simulink model "six_plus_six_AcmsteeringV09_main"  (R2014a)
settings: Solver=FixedStepDiscrete  StartTime=0.0  StopTime=10.0  FixedStep=0.0005  RelTol=1e-3
InitFcn:
  | Veh_Par_wxt
values from neighbouring files (symbols this model uses):
  acc_spdctl = [0 100]    [Veh_Par_wxt.m]
  ag_thr = ecucoder_cal(ag_thr)    [Veh_Par_wxt.m]
  B = 1.8    [Veh_Par_wxt.m]
  bra_em = 100    [Veh_Par_wxt.m]
  bra_pre_gz2 = 100/3    (= 33.3333333333)    [Veh_Par_wxt.m]
  bra_pre_gz34 = 10/3    (= 3.33333333333)    [Veh_Par_wxt.m]
  bra_pre_yd = 10/2    (= 5)    [Veh_Par_wxt.m]
  brakepre_dem_data = [0 1 2 3 4 5 6 7 8 9 10]    [Veh_Par_wxt.m]
  brakeTrq_dem_data = [0 125 251 376 502 627 753 878 1004 1129 1255]    [Veh_Par_wxt.m]
  bratrq_max = 4*1255    (= 5020)    [Veh_Par_wxt.m]
  eff_tran = 0.9    [Veh_Par_wxt.m]
  ESP_switch = ecucoder_cal(ESP_switch)    [Veh_Par_wxt.m]
  G = Mass*g    (= 15696)    [Veh_Par_wxt.m]
  kd1 = ecucoder_cal(kd1)    [Veh_Par_wxt.m]
  kd2 = 0    [Veh_Par_wxt.m]
  ki1 = ecucoder_cal(ki1)    [Veh_Par_wxt.m]
  ki2 = 1    [Veh_Par_wxt.m]
  kp1 = ecucoder_cal(kp1)    [Veh_Par_wxt.m]
  kp2 = 300    [Veh_Par_wxt.m]
  L = L1+L2    (= 2.9)    [Veh_Par_wxt.m]
  premax = 100    [Veh_Par_wxt.m]
  Radius = 0.4572/2    (= 0.2286)    [Veh_Par_wxt.m]
  RC_switch = ecucoder_cal(RC_switch)    [Veh_Par_wxt.m]
  s_opt_yi = 0.15    [Veh_Par_wxt.m]
  s_opt_zhuan = 0.8    [Veh_Par_wxt.m]
  s_opt_zhuan_add = 0.05    [Veh_Par_wxt.m]
  s_opt_zhuan_table = [0.8 0.8 0.3 0.3]    [Veh_Par_wxt.m]
  spd_map_mot = [0 499.85 999.79 1500 2000 2500 3000 3500 4000 4500 4999.8 5999.8]    [Veh_Par_wxt.m]
  spd_spdctl = [0 500]    [Veh_Par_wxt.m]
  speed_thr_park = 5/3.6/Radius*tras_ratio*30/pi    (= 464.143899364)    [Veh_Par_wxt.m]
  TCS_switch = ecucoder_cal(TCS_switch)    [Veh_Par_wxt.m]
  tras_ratio = 8    [Veh_Par_wxt.m]
  trq_map_mot = [70.5 70.012 71.154 65.797 53.917 45.159 38.073 32.685 27.48 17.133 14.949 10.07]    [Veh_Par_wxt.m]
  trqmax_yd = 70.5    [Veh_Par_wxt.m]
  trqmax_zx = 70.5    [Veh_Par_wxt.m]
  trqmaxneg = -70.5    [Veh_Par_wxt.m]
  v_gain = 0.9    [Veh_Par_wxt.m]
  v_table = [0 5 20 100]    [Veh_Par_wxt.m]
  v_thr_park = 5    [Veh_Par_wxt.m]
  zhidong_bianmazhi = [-140000 750000]    [Veh_Par_wxt.m]
  zhidong_down = -140000    [Veh_Par_wxt.m]
  zhidong_up = 750000    [Veh_Par_wxt.m]
  zhidong_youmen = [0 100]    [Veh_Par_wxt.m]
  zhuanxiang_bianmazhi = [-400000 0 400000]    [Veh_Par_wxt.m]
  zhuanxiang_down = -400000    [Veh_Par_wxt.m]
  zhuanxiang_up = 400000    [Veh_Par_wxt.m]
  zhuanxiang_youmen = [-100 0 100]    [Veh_Par_wxt.m]
undefined symbols (not defined in the file or in its folder): ecucoder_acal, guzhang_lf, guzhang_lm, guzhang_lr, guzhang_rf, guzhang_rm, guzhang_rr, myFIS
libraries: simulink x979, ec5744lib x59, fuzblock x2
(part 3 of 26)

== system six_plus_six_AcmsteeringV09_main/Data_input/MCU2 ==
  In1 : Inport
  In2 : Inport  Port=2
  Trigger : TriggerPort  TriggerType=function-call  PortDimensions=1
  MCU2 : Subsystem
  MCU2_MotorStallingFault : Outport
  MCU2_UdcDetectionFault : Outport  Port=2
  MCU2_TempSensorFault : Outport  Port=3
  MCU2_ActiveDischargingFault : Outport  Port=4
  MCU2_ldcSensorFault : Outport  Port=5
  MCU2_luSensorFault : Outport  Port=6
  MCU2_lvSensorFault : Outport  Port=7
  MCU2_FaultLevel : Outport  Port=8
  MCU2_Controllerload : Outport  Port=9
  MCU2_CanCommunicationFault : Outport  Port=10
  MCU2_MemoryFault : Outport  Port=11
  MCU2_DownratingFault : Outport  Port=12
  MCU2_IGBTFault : Outport  Port=13
  MCU2_MotorOverTemp : Outport  Port=14
  MCU2_ControllerOverTemp : Outport  Port=15
  MCU2_MotorOverSpeed : Outport  Port=16
  MCU2_RotaryInverterFault : Outport  Port=17
  MCU2_UnderVoltage : Outport  Port=18
  MCU2_OverVoltage : Outport  Port=19
  MCU2_MotorOverLoad : Outport  Port=20
  wires:
  MCU2/1(MCU2_MotorStallingFault_Out) -> MCU2_MotorStallingFault/1
  MCU2/7(MCU2_IvSensorFault_Out) -> MCU2_lvSensorFault/1
  MCU2/4(MCU2_ActieDischargingFault_Out) -> MCU2_ActiveDischargingFault/1
  MCU2/12(MCU2_DownratingFault_Out) -> MCU2_DownratingFault/1
  MCU2/13(MCU2_IGBTFault_Out) -> MCU2_IGBTFault/1
  MCU2/3(MCU2_TempSensorFault_Out) -> MCU2_TempSensorFault/1
  MCU2/10(MCU2_CanCommunicationFault_Out) -> MCU2_CanCommunicationFault/1
  MCU2/11(MCU2_MemoryFault_Out) -> MCU2_MemoryFault/1
  MCU2/14(MCU2_MotorOverTemp_Out) -> MCU2_MotorOverTemp/1
  MCU2/2(MCU2_UdcDetectionFault_Out) -> MCU2_UdcDetectionFault/1
  MCU2/5(MCU2_IdcSensorFault_Out) -> MCU2_ldcSensorFault/1
  In2/1 -> MCU2/1(input)
  In1/1 -> MCU2/Enable
  MCU2/6(MCU2_IuSensorFault_Out) -> MCU2_luSensorFault/1
  MCU2/8(MCU2_FaultLevel_Out) -> MCU2_FaultLevel/1
  MCU2/9(MCU2_ControllerOverload_Out) -> MCU2_Controllerload/1
  MCU2/20(MCU2_MotorOverLoad_Out) -> MCU2_MotorOverLoad/1
  MCU2/18(MCU2_UnderVoltage_Out) -> MCU2_UnderVoltage/1
  MCU2/19(MCU2_OverVoltage_Out) -> MCU2_OverVoltage/1
  MCU2/15(MCU2_ControllerOverTemp_Out) -> MCU2_ControllerOverTemp/1
  MCU2/16(MCU2_MotorOverSpeed_Out) -> MCU2_MotorOverSpeed/1
  MCU2/17(MCU2_RotaryInverterFault_Out) -> MCU2_RotaryInverterFault/1

== matlab function six_plus_six_AcmsteeringV09_main/Data_input/3/Enabled Subsystem/MATLAB Function1 ==
  data: current_in input; current_out output
function current_out = motec_current(current_in)
    if current_in>32768
        current_out=current_in-65535;
    else
        current_out=current_in;
    end
end

== matlab function six_plus_six_AcmsteeringV09_main/MainControl/mode_control/backward/backward/Brake/HeartBeat2 ==
  data: life_pre input; life output
function life = fcn(life_pre)
%#codegen
life=single(life_pre+1);
if life>255
    life=single(0);
end
end

== matlab function six_plus_six_AcmsteeringV09_main/MainControl/mode_control/backward/backward/Drive/左右侧电机分配及功率限制/MATLAB Function ==
  data: trqlim_l input; trq_dem_l output; trq_dem_r output; trq_dem_l1 input; trqlim_r input; trq_dem_r1 input; delta_T_dem input
function [trq_dem_l,trq_dem_r] = fcn(trqlim_l,trq_dem_l1,trqlim_r,trq_dem_r1,delta_T_dem)
%#codegen
if trq_dem_l1==trqlim_l
    trq_dem_l=single(trq_dem_l1);
    trq_dem_r=single(trq_dem_l1+delta_T_dem);%这时候加的是负值
elseif trq_dem_r1==trqlim_r
    trq_dem_l=single(trq_dem_r1-delta_T_dem);
    trq_dem_r=single(trq_dem_r1);
    
else
    trq_dem_l=single(trq_dem_l1);
    trq_dem_r=single(trq_dem_r1);
end
% trq_dem_l=single(max(0,trq_dem_l));%限一下最小值，不要小于0
% trq_dem_r=single(max(0,trq_dem_r));
trq_dem_l=single(max(-trqlim_l,trq_dem_l));%小转向半径下，内侧履带是可能输出负转矩的，从地面吸收功率，给外侧，所以不能限到0，限到最大电机外特性负值
trq_dem_r=single(max(-trqlim_r,trq_dem_r));
end

== matlab function six_plus_six_AcmsteeringV09_main/MainControl/mode_control/forward/forward/Brake/HeartBeat ==
  data: life_pre input; life output
function life = fcn(life_pre)
%#codegen
life=single(life_pre+1);
if life>255
    life=single(0);
end
end

== matlab function six_plus_six_AcmsteeringV09_main/MainControl/mode_control/center_steer/center_steer/HeartBeat4 ==
  data: life_pre input; life output
function life = fcn(life_pre)
%#codegen
life=single(life_pre+1);
if life>255
    life=single(0);
end
end

== matlab function six_plus_six_AcmsteeringV09_main/MainControl/mode_control/emergency_stop/emergency_stop/HeartBeat5 ==
  data: life_pre input; life output
function life = fcn(life_pre)
%#codegen
life=single(life_pre+1);
if life>255
    life=single(0);
end
end

== matlab function six_plus_six_AcmsteeringV09_main/MainControl/mode_control/neutral/neutral/HeartBeat5 ==
  data: life_pre input; life output
function life = fcn(life_pre)
%#codegen
life=single(life_pre+1);
if life>255
    life=single(0);
end
end

== matlab function six_plus_six_AcmsteeringV09_main/MainControl/mode_control/backward/backward/Drive/驱动防滑控制TCS/直行TCS/直行/MATLAB Function2 ==
  data: s_act_rf input; flag_rf output; s_opt_zhuan input; s_opt_zhuan_add input; flag_rf_pre input int8
function flag_rf = fcn(s_act_rf,s_opt_zhuan,s_opt_zhuan_add,flag_rf_pre)
%#codegen
if s_act_rf>s_opt_zhuan+s_opt_zhuan_add
    flag_rf=int8(1);
elseif s_act_rf<s_opt_zhuan
    flag_rf =int8(0);
else
    flag_rf=int8(flag_rf_pre);
end
end

== matlab function six_plus_six_AcmsteeringV09_main/Data_input/5/Enabled Subsystem/MATLAB Function ==
  data: data1 input; y output; data2 input; data3 input; data4 input
function y = fcn(data1,data2,data3,data4)
%#codegen
y1=data4*256^3+data3*256^2+data2*256+data1;
y=typecast(uint32(y1),'single');
end
% y = u;

== matlab function six_plus_six_AcmsteeringV09_main/Data_input/7/Enabled
Subsystem/MATLAB Function1 ==
  data: data1 input; y output; data2 input; data3 input; data4 input
function y = fcn(data1,data2,data3,data4)
%#codegen
y1=data4*256^3+data3*256^2+data2*256+data1;
y=typecast(uint32(y1),'single');
end
% y = u;

== matlab function six_plus_six_AcmsteeringV09_main/InputSignalProcess/MATLAB Function1 ==
  data: Xangularrate input; Yangularrate input; Zangularrate input; Xacceleration input; Yacceleration input; Zacceleration input; Xangularrate1 output; Yangularrate1 output; Zangularrate1 output; Xacceleration1 output; Yacceleration1 output; Zacceleration1 output; NorthSpd1 output; SkySpd1 output; EastSpd1 output; Altitude1 output; Longitude1 output; Latitude1 output; Rolling1 output; Heading1 output; Pitching1 output; NorthSpd input; SkySpd input; Xspd output; EastSpd input; Altitude input; Longitude input; Latitude input; Rolling input; Heading input; Yspd output; Pitching input
function [Xangularrate1,Yangularrate1,Zangularrate1,Xacceleration1,Yacceleration1,Zacceleration1,NorthSpd1,SkySpd1,EastSpd1,Altitude1,Longitude1,Latitude1,Rolling1,Heading1,Pitching1,Xspd,Yspd] = fcn(Xangularrate,Yangularrate,Zangularrate,Xacceleration,Yacceleration,Zacceleration,NorthSpd,SkySpd,EastSpd,Altitude,Longitude,Latitude,Rolling,Heading,Pitching)
%#codegen
Xangularrate1=Xangularrate;
Yangularrate1=-Zangularrate;
Zangularrate1=-Yangularrate;
Xacceleration1=Xacceleration;
Yacceleration1=-Zacceleration;
Zacceleration1=-Yacceleration;
NorthSpd1=NorthSpd;
SkySpd1=SkySpd;
EastSpd1=EastSpd;
Altitude1=Altitude;
Longitude1=Longitude;
Latitude1=Latitude;
Rolling1=Rolling;
Heading1=Heading;
Pitching1=Pitching;
Xspd=NorthSpd*cos(Heading/180*pi)-EastSpd*sin(Heading/180*pi);
Yspd=-(NorthSpd*sin(Heading/180*pi)+EastSpd*cos(Heading/180*pi));
end
% y = u;

== system six_plus_six_AcmsteeringV09_main/Data_input/MCU2_1 ==
  In1 : Inport
  In2 : Inport  Port=2
  Trigger : TriggerPort  TriggerType=function-call  PortDimensions=1
  MCU2 : Subsystem
  MCU2_MotorStallingFault : Outport
  MCU2_UdcDetectionFault : Outport  Port=2
  MCU2_TempSensorFault : Outport  Port=3
  MCU2_ActiveDischargingFault : Outport  Port=4
  MCU2_ldcSensorFault : Outport  Port=5
  MCU2_luSensorFault : Outport  Port=6
  MCU2_lvSensorFault : Outport  Port=7
  MCU2_FaultLevel : Outport  Port=8
  MCU2_Controllerload : Outport  Port=9
  MCU2_CanCommunicationFault : Outport  Port=10
  MCU2_MemoryFault : Outport  Port=11
  MCU2_DownratingFault : Outport  Port=12
  MCU2_IGBTFault : Outport  Port=13
  MCU2_MotorOverTemp : Outport  Port=14
  MCU2_ControllerOverTemp : Outport  Port=15
  MCU2_MotorOverSpeed : Outport  Port=16
  MCU2_RotaryInverterFault : Outport  Port=17
  MCU2_UnderVoltage : Outport  Port=18
  MCU2_OverVoltage : Outport  Port=19
  MCU2_MotorOverLoad : Outport  Port=20
  wires:
  MCU2/1(MCU2_MotorStallingFault_Out) -> MCU2_MotorStallingFault/1
  MCU2/7(MCU2_IvSensorFault_Out) -> MCU2_lvSensorFault/1
  MCU2/4(MCU2_ActieDischargingFault_Out) -> MCU2_ActiveDischargingFault/1
  MCU2/12(MCU2_DownratingFault_Out) -> MCU2_DownratingFault/1
  MCU2/13(MCU2_IGBTFault_Out) -> MCU2_IGBTFault/1
  MCU2/3(MCU2_TempSensorFault_Out) -> MCU2_TempSensorFault/1
  MCU2/10(MCU2_CanCommunicationFault_Out) -> MCU2_CanCommunicationFault/1
  MCU2/11(MCU2_MemoryFault_Out) -> MCU2_MemoryFault/1
  MCU2/14(MCU2_MotorOverTemp_Out) -> MCU2_MotorOverTemp/1
  MCU2/2(MCU2_UdcDetectionFault_Out) -> MCU2_UdcDetectionFault/1
  MCU2/5(MCU2_IdcSensorFault_Out) -> MCU2_ldcSensorFault/1
  In2/1 -> MCU2/1(input)
  In1/1 -> MCU2/Enable
  MCU2/6(MCU2_IuSensorFault_Out) -> MCU2_luSensorFault/1
  MCU2/8(MCU2_FaultLevel_Out) -> MCU2_FaultLevel/1
  MCU2/9(MCU2_ControllerOverload_Out) -> MCU2_Controllerload/1
  MCU2/20(MCU2_MotorOverLoad_Out) -> MCU2_MotorOverLoad/1
  MCU2/18(MCU2_UnderVoltage_Out) -> MCU2_UnderVoltage/1
  MCU2/19(MCU2_OverVoltage_Out) -> MCU2_OverVoltage/1
  MCU2/15(MCU2_ControllerOverTemp_Out) -> MCU2_ControllerOverTemp/1
  MCU2/16(MCU2_MotorOverSpeed_Out) -> MCU2_MotorOverSpeed/1
  MCU2/17(MCU2_RotaryInverterFault_Out) -> MCU2_RotaryInverterFault/1

== system six_plus_six_AcmsteeringV09_main/Data_input/MCU2_2 ==
  In1 : Inport
  In2 : Inport  Port=2
  Trigger : TriggerPort  TriggerType=function-call  PortDimensions=1
  MCU2 : Subsystem
  MCU2_MotorStallingFault : Outport
  MCU2_UdcDetectionFault : Outport  Port=2
  MCU2_TempSensorFault : Outport  Port=3
  MCU2_ActiveDischargingFault : Outport  Port=4
  MCU2_ldcSensorFault : Outport  Port=5
  MCU2_luSensorFault : Outport  Port=6
  MCU2_lvSensorFault : Outport  Port=7
  MCU2_FaultLevel : Outport  Port=8
  MCU2_Controllerload : Outport  Port=9
  MCU2_CanCommunicationFault : Outport  Port=10
  MCU2_MemoryFault : Outport  Port=11
  MCU2_DownratingFault : Outport  Port=12
  MCU2_IGBTFault : Outport  Port=13
  MCU2_MotorOverTemp : Outport  Port=14
  MCU2_ControllerOverTemp : Outport  Port=15
  MCU2_MotorOverSpeed : Outport  Port=16
  MCU2_RotaryInverterFault : Outport  Port=17
  MCU2_UnderVoltage : Outport  Port=18
  MCU2_OverVoltage : Outport  Port=19
  MCU2_MotorOverLoad : Outport  Port=20
  wires:
  MCU2/1(MCU2_MotorStallingFault_Out) -> MCU2_MotorStallingFault/1
  MCU2/7(MCU2_IvSensorFault_Out) -> MCU2_lvSensorFault/1
  MCU2/4(MCU2_ActieDischargingFault_Out) -> MCU2_ActiveDischargingFault/1
  MCU2/12(MCU2_DownratingFault_Out) -> MCU2_DownratingFault/1
  MCU2/13(MCU2_IGBTFault_Out) -> MCU2_IGBTFault/1
  MCU2/3(MCU2_TempSensorFault_Out) -> MCU2_TempSensorFault/1
  MCU2/10(MCU2_CanCommunicationFault_Out) -> MCU2_CanCommunicationFault/1
  MCU2/11(MCU2_MemoryFault_Out) -> MCU2_MemoryFault/1
  MCU2/14(MCU2_MotorOverTemp_Out) -> MCU2_MotorOverTemp/1
  MCU2/2(MCU2_UdcDetectionFault_Out) -> MCU2_UdcDetectionFault/1
  MCU2/5(MCU2_IdcSensorFault_Out) -> MCU2_ldcSensorFault/1
  In2/1 -> MCU2/1(input)
  In1/1 -> MCU2/Enable
  MCU2/6(MCU2_IuSensorFault_Out) -> MCU2_luSensorFault/1
  MCU2/8(MCU2_FaultLevel_Out) -> MCU2_FaultLevel/1
  MCU2/9(MCU2_ControllerOverload_Out) -> MCU2_Controllerload/1
  MCU2/20(MCU2_MotorOverLoad_Out) -> MCU2_MotorOverLoad/1
  MCU2/18(MCU2_UnderVoltage_Out) -> MCU2_UnderVoltage/1
  MCU2/19(MCU2_OverVoltage_Out) -> MCU2_OverVoltage/1
  MCU2/15(MCU2_ControllerOverTemp_Out) -> MCU2_ControllerOverTemp/1
  MCU2/16(MCU2_MotorOverSpeed_Out) -> MCU2_MotorOverSpeed/1
  MCU2/17(MCU2_RotaryInverterFault_Out) -> MCU2_RotaryInverterFault/1

== system six_plus_six_AcmsteeringV09_main/Data_input/MCU2_3 ==
  In1 : Inport
  In2 : Inport  Port=2
  Trigger : TriggerPort  TriggerType=function-call  PortDimensions=1
  MCU2 : Subsystem
  MCU2_MotorStallingFault : Outport
  MCU2_UdcDetectionFault : Outport  Port=2
  MCU2_TempSensorFault : Outport  Port=3
  MCU2_ActiveDischargingFault : Outport  Port=4
  MCU2_ldcSensorFault : Outport  Port=5
  MCU2_luSensorFault : Outport  Port=6
  MCU2_lvSensorFault : Outport  Port=7
  MCU2_FaultLevel : Outport  Port=8
  MCU2_Controllerload : Outport  Port=9
  MCU2_CanCommunicationFault : Outport  Port=10
  MCU2_MemoryFault : Outport  Port=11
  MCU2_DownratingFault : Outport  Port=12
  MCU2_IGBTFault : Outport  Port=13
  MCU2_MotorOverTemp : Outport  Port=14
  MCU2_ControllerOverTemp : Outport  Port=15
  MCU2_MotorOverSpeed : Outport  Port=16
  MCU2_RotaryInverterFault : Outport  Port=17
  MCU2_UnderVoltage : Outport  Port=18
  MCU2_OverVoltage : Outport  Port=19
  MCU2_MotorOverLoad : Outport  Port=20
  wires:
  MCU2/1(MCU2_MotorStallingFault_Out) -> MCU2_MotorStallingFault/1
  MCU2/7(MCU2_IvSensorFault_Out) -> MCU2_lvSensorFault/1
  MCU2/4(MCU2_ActieDischargingFault_Out) -> MCU2_ActiveDischargingFault/1
  MCU2/12(MCU2_DownratingFault_Out) -> MCU2_DownratingFault/1
  MCU2/13(MCU2_IGBTFault_Out) -> MCU2_IGBTFault/1
  MCU2/3(MCU2_TempSensorFault_Out) -> MCU2_TempSensorFault/1
  MCU2/10(MCU2_CanCommunicationFault_Out) -> MCU2_CanCommunicationFault/1
  MCU2/11(MCU2_MemoryFault_Out) -> MCU2_MemoryFault/1
  MCU2/14(MCU2_MotorOverTemp_Out) -> MCU2_MotorOverTemp/1
  MCU2/2(MCU2_UdcDetectionFault_Out) -> MCU2_UdcDetectionFault/1
  MCU2/5(MCU2_IdcSensorFault_Out) -> MCU2_ldcSensorFault/1
  In2/1 -> MCU2/1(input)
  In1/1 -> MCU2/Enable
  MCU2/6(MCU2_IuSensorFault_Out) -> MCU2_luSensorFault/1
  MCU2/8(MCU2_FaultLevel_Out) -> MCU2_FaultLevel/1
  MCU2/9(MCU2_ControllerOverload_Out) -> MCU2_Controllerload/1
  MCU2/20(MCU2_MotorOverLoad_Out) -> MCU2_MotorOverLoad/1
  MCU2/18(MCU2_UnderVoltage_Out) -> MCU2_UnderVoltage/1
  MCU2/19(MCU2_OverVoltage_Out) -> MCU2_OverVoltage/1
  MCU2/15(MCU2_ControllerOverTemp_Out) -> MCU2_ControllerOverTemp/1
  MCU2/16(MCU2_MotorOverSpeed_Out) -> MCU2_MotorOverSpeed/1
  MCU2/17(MCU2_RotaryInverterFault_Out) -> MCU2_RotaryInverterFault/1

== system six_plus_six_AcmsteeringV09_main/Data_input/MCU2_4 ==
  In1 : Inport
  In2 : Inport  Port=2
  Trigger : TriggerPort  TriggerType=function-call  PortDimensions=1
  MCU2 : Subsystem
  MCU2_MotorStallingFault : Outport
  MCU2_UdcDetectionFault : Outport  Port=2
  MCU2_TempSensorFault : Outport  Port=3
  MCU2_ActiveDischargingFault : Outport  Port=4
  MCU2_ldcSensorFault : Outport  Port=5
  MCU2_luSensorFault : Outport  Port=6
  MCU2_lvSensorFault : Outport  Port=7
  MCU2_FaultLevel : Outport  Port=8
  MCU2_Controllerload : Outport  Port=9
  MCU2_CanCommunicationFault : Outport  Port=10
  MCU2_MemoryFault : Outport  Port=11
  MCU2_DownratingFault : Outport  Port=12
  MCU2_IGBTFault : Outport  Port=13
  MCU2_MotorOverTemp : Outport  Port=14
  MCU2_ControllerOverTemp : Outport  Port=15
  MCU2_MotorOverSpeed : Outport  Port=16
  MCU2_RotaryInverterFault : Outport  Port=17
  MCU2_UnderVoltage : Outport  Port=18
  MCU2_OverVoltage : Outport  Port=19
  MCU2_MotorOverLoad : Outport  Port=20
  wires:
  MCU2/1(MCU2_MotorStallingFault_Out) -> MCU2_MotorStallingFault/1
  MCU2/7(MCU2_IvSensorFault_Out) -> MCU2_lvSensorFault/1
  MCU2/4(MCU2_ActieDischargingFault_Out) -> MCU2_ActiveDischargingFault/1
  MCU2/12(MCU2_DownratingFault_Out) -> MCU2_DownratingFault/1
  MCU2/13(MCU2_IGBTFault_Out) -> MCU2_IGBTFault/1
  MCU2/3(MCU2_TempSensorFault_Out) -> MCU2_TempSensorFault/1
  MCU2/10(MCU2_CanCommunicationFault_Out) -> MCU2_CanCommunicationFault/1
  MCU2/11(MCU2_MemoryFault_Out) -> MCU2_MemoryFault/1
  MCU2/14(MCU2_MotorOverTemp_Out) -> MCU2_MotorOverTemp/1
  MCU2/2(MCU2_UdcDetectionFault_Out) -> MCU2_UdcDetectionFault/1
  MCU2/5(MCU2_IdcSensorFault_Out) -> MCU2_ldcSensorFault/1
  In2/1 -> MCU2/1(input)
  In1/1 -> MCU2/Enable
  MCU2/6(MCU2_IuSensorFault_Out) -> MCU2_luSensorFault/1
  MCU2/8(MCU2_FaultLevel_Out) -> MCU2_FaultLevel/1
  MCU2/9(MCU2_ControllerOverload_Out) -> MCU2_Controllerload/1
  MCU2/20(MCU2_MotorOverLoad_Out) -> MCU2_MotorOverLoad/1
  MCU2/18(MCU2_UnderVoltage_Out) -> MCU2_UnderVoltage/1
  MCU2/19(MCU2_OverVoltage_Out) -> MCU2_OverVoltage/1
  MCU2/15(MCU2_ControllerOverTemp_Out) -> MCU2_ControllerOverTemp/1
  MCU2/16(MCU2_MotorOverSpeed_Out) -> MCU2_MotorOverSpeed/1
  MCU2/17(MCU2_RotaryInverterFault_Out) -> MCU2_RotaryInverterFault/1

== system six_plus_six_AcmsteeringV09_main/Data_input/MCU2_5 ==
  In1 : Inport
  In2 : Inport  Port=2
  Trigger : TriggerPort  TriggerType=function-call  PortDimensions=1
  MCU2 : Subsystem
  MCU2_MotorStallingFault : Outport
  MCU2_UdcDetectionFault : Outport  Port=2
  MCU2_TempSensorFault : Outport  Port=3
  MCU2_ActiveDischargingFault : Outport  Port=4
  MCU2_ldcSensorFault : Outport  Port=5
  MCU2_luSensorFault : Outport  Port=6
  MCU2_lvSensorFault : Outport  Port=7
  MCU2_FaultLevel : Outport  Port=8
  MCU2_Controllerload : Outport  Port=9
  MCU2_CanCommunicationFault : Outport  Port=10
  MCU2_MemoryFault : Outport  Port=11
  MCU2_DownratingFault : Outport  Port=12
  MCU2_IGBTFault : Outport  Port=13
  MCU2_MotorOverTemp : Outport  Port=14
  MCU2_ControllerOverTemp : Outport  Port=15
  MCU2_MotorOverSpeed : Outport  Port=16
  MCU2_RotaryInverterFault : Outport  Port=17
  MCU2_UnderVoltage : Outport  Port=18
  MCU2_OverVoltage : Outport  Port=19
  MCU2_MotorOverLoad : Outport  Port=20
  wires:
  MCU2/1(MCU2_MotorStallingFault_Out) -> MCU2_MotorStallingFault/1
  MCU2/7(MCU2_IvSensorFault_Out) -> MCU2_lvSensorFault/1
  MCU2/4(MCU2_ActieDischargingFault_Out) -> MCU2_ActiveDischargingFault/1
  MCU2/12(MCU2_DownratingFault_Out) -> MCU2_DownratingFault/1
  MCU2/13(MCU2_IGBTFault_Out) -> MCU2_IGBTFault/1
  MCU2/3(MCU2_TempSensorFault_Out) -> MCU2_TempSensorFault/1
  MCU2/10(MCU2_CanCommunicationFault_Out) -> MCU2_CanCommunicationFault/1
  MCU2/11(MCU2_MemoryFault_Out) -> MCU2_MemoryFault/1
  MCU2/14(MCU2_MotorOverTemp_Out) -> MCU2_MotorOverTemp/1
  MCU2/2(MCU2_UdcDetectionFault_Out) -> MCU2_UdcDetectionFault/1
  MCU2/5(MCU2_IdcSensorFault_Out) -> MCU2_ldcSensorFault/1
  In2/1 -> MCU2/1(input)
  In1/1 -> MCU2/Enable
  MCU2/6(MCU2_IuSensorFault_Out) -> MCU2_luSensorFault/1
  MCU2/8(MCU2_FaultLevel_Out) -> MCU2_FaultLevel/1
  MCU2/9(MCU2_ControllerOverload_Out) -> MCU2_Controllerload/1
  MCU2/20(MCU2_MotorOverLoad_Out) -> MCU2_MotorOverLoad/1
  MCU2/18(MCU2_UnderVoltage_Out) -> MCU2_UnderVoltage/1
  MCU2/19(MCU2_OverVoltage_Out) -> MCU2_OverVoltage/1
  MCU2/15(MCU2_ControllerOverTemp_Out) -> MCU2_ControllerOverTemp/1
  MCU2/16(MCU2_MotorOverSpeed_Out) -> MCU2_MotorOverSpeed/1
  MCU2/17(MCU2_RotaryInverterFault_Out) -> MCU2_RotaryInverterFault/1

== system six_plus_six_AcmsteeringV09_main/Data_input/RemoteControl1 ==
  In1 : Inport
  In2 : Inport  Port=2
  Trigger : TriggerPort  TriggerType=function-call  PortDimensions=1
  Yaokong2 : Subsystem
  SH : Outport
  SE : Outport  Port=2
  SD : Outport  Port=3
  SA : Outport  Port=4
  LIFEspan : Outport  Port=5
  wires:
  Yaokong2/2(SE_Out) -> SE/1
  Yaokong2/3(SD_Out) -> SD/1
  Yaokong2/4(SA_Out) -> SA/1
  In2/1 -> Yaokong2/1(input)
  In1/1 -> Yaokong2/Enable
  Yaokong2/1(SH_Out) -> SH/1
  Yaokong2/5(LIFEspan_Out) -> LIFEspan/1

== system six_plus_six_AcmsteeringV09_main/Data_input/RemoteControl2 ==
  In1 : Inport
  In2 : Inport  Port=2
  Trigger : TriggerPort  TriggerType=function-call  PortDimensions=1
  Yaokong1 : Subsystem
  Rightstick_updown : Outport
  Rightstick_leftright : Outport  Port=2
  Leftstick_updown : Outport  Port=3
  Leftstick_leftright : Outport  Port=4
  wires:
  In1/1 -> Yaokong1/Enable
  In2/1 -> Yaokong1/1(input)
  Yaokong1/1(Rightstick_updown_Out) -> Rightstick_updown/1
  Yaokong1/2(Rightstick_leftright_Out) -> Rightstick_leftright/1
  Yaokong1/3(Leftstick_updown_Out) -> Leftstick_updown/1
  Yaokong1/4(Leftstick_leftright_Out) -> Leftstick_leftright/1

== system six_plus_six_AcmsteeringV09_main/MainControl/mode_control ==
  mode_dem_out : Inport
  Signals : Inport  Port=2
  Multiport Switch : MultiPortSwitch  DataPortOrder=Zero-based contiguous  Inputs=6
  Park : Subsystem  TreatAsAtomicUnit=on
  Switch Case : SwitchCase  CaseConditions={0,1,2,3,4,5}  ShowDefaultCase=off
  backward : Subsystem  TreatAsAtomicUnit=on
  center_steer : Subsystem  TreatAsAtomicUnit=on
  emergency_stop : Subsystem  TreatAsAtomicUnit=on
  forward : Subsystem  TreatAsAtomicUnit=on
  neutral : Subsystem  TreatAsAtomicUnit=on
  com_dem : Outport
  wires:
  mode_dem_out/1 -> Multiport Switch/1, Switch Case/1
  Signals/1 -> backward/1(Signals), emergency_stop/1(Signals), center_steer/1(Signals), neutral/1(Signals), forward/1(Signals), Park/1(Signals)
  Switch Case/1 -> Park/Action
  Switch Case/6 -> emergency_stop/Action
  Switch Case/5 -> center_steer/Action
  Switch Case/4 -> backward/Action
  Switch Case/3 -> neutral/Action
  Switch Case/2 -> forward/Action
  Park/1(park_dem) -> Multiport Switch/2
  forward/1(forward_dem) -> Multiport Switch/3
  backward/1(backward_dem) -> Multiport Switch/5
  neutral/1(neutral_dem) -> Multiport Switch/4
  center_steer/1(center_steer_dem) -> Multiport Switch/6
  emergency_stop/1(emergency_stop_dem) -> Multiport Switch/7
  Multiport Switch/1 -> com_dem/1

== system six_plus_six_AcmsteeringV09_main/MainControl/mode_switch ==
  Signals : Inport
  Abs{,1..5} (6 alike) : Abs  OutDataTypeStr=single
  Bus Selector : BusSelector  OutputSignals=RemoteControl_dem.brake_emerg,RemoteControl_dem.park,RemoteControl_dem.acc_dem,RemoteControl_dem.steer_dem,RemoteControl_dem.brake_dem,RemoteControl_dem.center,MOTOR.MOTOR1.MCU0.MCU0_SpeedFdk,MOTOR.MOTOR2.MCU0_1.MCU0_1SpeedFdk,MOTOR.MOTOR3.MCU0_2.MCU0_2SpeedFdk,MOTOR.MOTOR4.MCU0_3.MCU0_3SpeedFdk,MOTOR.MOTOR5.MCU0_4.MCU0_4SpeedFdk,MOTOR.MOTOR6.MCU0_5.MCU0_5SpeedFdk
  Constant1 : Constant  Value=v_thr_park  OutDataTypeStr=single  SampleTime=-1
  Constant2 : Constant  Value=speed_thr_park  OutDataTypeStr=single  SampleTime=-1
  Memory : Memory  InheritSampleTime=on
  Terminator : Terminator
  mode_switch : MATLAB Function  TreatAsAtomicUnit=on
  mode_dem_out : Outport
  wires:
  Memory/1 -> mode_switch/14(mode_dem_out_pre)
  Signals/1 -> Bus Selector/1
  Constant2/1 -> mode_switch/13(speed_thr_park)
  mode_switch/1(mode_dem_out) -> Memory/1, mode_dem_out/1  "mode_dem_out"
  Bus Selector/1 -> mode_switch/1(brake_emerg)  "<brake_emerg>"
  Bus Selector/2 -> mode_switch/2(park)  "<park>"
  Bus Selector/3 -> mode_switch/3(acc_dem)  "<acc_dem>"
  Bus Selector/4 -> mode_switch/4(steer_dem)  "<steer_dem>"
  Bus Selector/5 -> mode_switch/5(brake_dem)  "<brake_dem>"
  Bus Selector/7 -> Abs/1  "<MCU0_SpeedFdk>"
  Bus Selector/8 -> Abs1/1  "<MCU0_1SpeedFdk>"
  Bus Selector/9 -> Abs2/1  "<MCU0_2SpeedFdk>"
  Bus Selector/10 -> Abs3/1  "<MCU0_3SpeedFdk>"
  Bus Selector/11 -> Abs4/1  "<MCU0_4SpeedFdk>"
  Bus Selector/12 -> Abs5/1  "<MCU0_5SpeedFdk>"
  Abs/1 -> mode_switch/7(MCU0_SpeedFdk)
  Abs1/1 -> mode_switch/8(MCU0_1SpeedFdk)
  Abs2/1 -> mode_switch/9(MCU0_2SpeedFdk)
  Abs3/1 -> mode_switch/10(MCU0_3SpeedFdk)
  Abs4/1 -> mode_switch/11(MCU0_4SpeedFdk)
  Abs5/1 -> mode_switch/12(MCU0_5SpeedFdk)
  Constant1/1 -> Terminator/1
  Bus Selector/6 -> mode_switch/6(center)  "<center>"

== system six_plus_six_AcmsteeringV09_main/Subsystem/VCU1 ==
  VCU1_EnableReq_in : Inport
  VCU1_CtrlModel_in : Inport  Port=2
  VCU1_GearCmd_in : Inport  Port=3
  VCU1_SpeedMax_in : Inport  Port=4
  VCU1_TorqueRef_in : Inport  Port=5
  VCU1_LifeCnt_in : Inport  Port=6
  Conv{1..8} (8 alike) : DataTypeConversion
  VCU1_CtrlModel : Subsystem
  VCU1_DLC : Constant  Value=8  OutDataTypeStr=uint8
  VCU1_DLC_Out : Terminator
  VCU1_EnableReq : Subsystem
  VCU1_GearCmd : Subsystem
  VCU1_ID : Constant  Value=2353065767  OutDataTypeStr=single
  VCU1_ID_Out : Terminator
  VCU1_LifeCnt : Subsystem
  VCU1_SpeedMax : Subsystem
  VCU1_TorqueRef : Subsystem
  VCU1_mux : Mux  Inputs=8
  or{1..8} (8 alike) : simulink/Logic and Bit Operations/Bitwise Operator  logicop=OR  UseBitMask=off  NumInputPorts=6  BitMask=bin2dec('11011001')  BitMaskRealWorld=Stored Integer
  output : Outport
  wires:
  VCU1_mux/1 -> output/1
  VCU1_LifeCnt/1(output1) -> or1/1
  VCU1_LifeCnt/2(output2) -> or2/1
  VCU1_LifeCnt/3(output3) -> or3/1
  VCU1_LifeCnt/4(output4) -> or4/1
  VCU1_LifeCnt/5(output5) -> or5/1
  VCU1_LifeCnt/6(output6) -> or6/1
  VCU1_LifeCnt/7(output7) -> or7/1
  VCU1_LifeCnt/8(output8) -> or8/1
  VCU1_TorqueRef/1(output1) -> or1/2
  VCU1_TorqueRef/2(output2) -> or2/2
  VCU1_TorqueRef/3(output3) -> or3/2
  VCU1_TorqueRef/4(output4) -> or4/2
  VCU1_TorqueRef/5(output5) -> or5/2
  VCU1_TorqueRef/6(output6) -> or6/2
  VCU1_TorqueRef/7(output7) -> or7/2
  VCU1_TorqueRef/8(output8) -> or8/2
  VCU1_SpeedMax/1(output1) -> or1/3
  VCU1_SpeedMax/2(output2) -> or2/3
  VCU1_SpeedMax/3(output3) -> or3/3
  VCU1_SpeedMax/4(output4) -> or4/3
  VCU1_SpeedMax/5(output5) -> or5/3
  VCU1_SpeedMax/6(output6) -> or6/3
  VCU1_SpeedMax/7(output7) -> or7/3
  VCU1_SpeedMax/8(output8) -> or8/3
  VCU1_GearCmd/1(output1) -> or1/4
  VCU1_GearCmd/2(output2) -> or2/4
  VCU1_GearCmd/3(output3) -> or3/4
  VCU1_GearCmd/4(output4) -> or4/4
  VCU1_GearCmd/5(output5) -> or5/4
  VCU1_GearCmd/6(output6) -> or6/4
  VCU1_GearCmd/7(output7) -> or7/4
  VCU1_GearCmd/8(output8) -> or8/4
  VCU1_CtrlModel/1(output1) -> or1/5
  VCU1_CtrlModel/2(output2) -> or2/5
  VCU1_CtrlModel/3(output3) -> or3/5
  VCU1_CtrlModel/4(output4) -> or4/5
  VCU1_CtrlModel/5(output5) -> or5/5
  VCU1_CtrlModel/6(output6) -> or6/5
  VCU1_CtrlModel/7(output7) -> or7/5
  VCU1_CtrlModel/8(output8) -> or8/5
  VCU1_EnableReq/1(output1) -> or1/6
  VCU1_EnableReq/2(output2) -> or2/6
  VCU1_EnableReq/3(output3) -> or3/6
  VCU1_EnableReq/4(output4) -> or4/6
  VCU1_EnableReq/5(output5) -> or5/6
  VCU1_EnableReq/6(output6) -> or6/6
  VCU1_EnableReq/7(output7) -> or7/6
  VCU1_EnableReq/8(output8) -> or8/6
  or1/1 -> Conv1/1
  Conv1/1 -> VCU1_mux/1
  or2/1 -> Conv2/1
  Conv2/1 -> VCU1_mux/2
  or3/1 -> Conv3/1
  Conv3/1 -> VCU1_mux/3
  or4/1 -> Conv4/1
  Conv4/1 -> VCU1_mux/4
  or5/1 -> Conv5/1
  Conv5/1 -> VCU1_mux/5
  or6/1 -> Conv6/1
  Conv6/1 -> VCU1_mux/6
  or7/1 -> Conv7/1
  Conv7/1 -> VCU1_mux/7
  or8/1 -> Conv8/1
  Conv8/1 -> VCU1_mux/8
  VCU1_ID/1 -> VCU1_ID_Out/1
  VCU1_DLC/1 -> VCU1_DLC_Out/1
  VCU1_LifeCnt_in/1 -> VCU1_LifeCnt/1(VCU1_LifeCnt)
  VCU1_TorqueRef_in/1 -> VCU1_TorqueRef/1(VCU1_TorqueRef)
  VCU1_SpeedMax_in/1 -> VCU1_SpeedMax/1(VCU1_SpeedMax)
  VCU1_GearCmd_in/1 -> VCU1_GearCmd/1(VCU1_GearCmd)
  VCU1_CtrlModel_in/1 -> VCU1_CtrlModel/1(VCU1_CtrlModel)
  VCU1_EnableReq_in/1 -> VCU1_EnableReq/1(VCU1_EnableReq)

== system six_plus_six_AcmsteeringV09_main/Subsystem/VCU2 ==
  VCU1_EnableReq_in : Inport
  VCU1_CtrlModel_in : Inport  Port=2
  VCU1_GearCmd_in : Inport  Port=3
  VCU1_SpeedMax_in : Inport  Port=4
  VCU1_TorqueRef_in : Inport  Port=5
  VCU1_LifeCnt_in : Inport  Port=6
  Conv{1..8} (8 alike) : DataTypeConversion
  VCU1_CtrlModel : Subsystem
  VCU1_DLC : Constant  Value=8  OutDataTypeStr=uint8
  VCU1_DLC_Out : Terminator
  VCU1_EnableReq : Subsystem
  VCU1_GearCmd : Subsystem
  VCU1_ID : Constant  Value=2353065767  OutDataTypeStr=single
  VCU1_ID_Out : Terminator
  VCU1_LifeCnt : Subsystem
  VCU1_SpeedMax : Subsystem
  VCU1_TorqueRef : Subsystem
  VCU1_mux : Mux  Inputs=8
  or{1..8} (8 alike) : simulink/Logic and Bit Operations/Bitwise Operator  logicop=OR  UseBitMask=off  NumInputPorts=6  BitMask=bin2dec('11011001')  BitMaskRealWorld=Stored Integer
  output : Outport
  wires:
  VCU1_mux/1 -> output/1
  VCU1_LifeCnt/1(output1) -> or1/1
  VCU1_LifeCnt/2(output2) -> or2/1
  VCU1_LifeCnt/3(output3) -> or3/1
  VCU1_LifeCnt/4(output4) -> or4/1
  VCU1_LifeCnt/5(output5) -> or5/1
  VCU1_LifeCnt/6(output6) -> or6/1
  VCU1_LifeCnt/7(output7) -> or7/1
  VCU1_LifeCnt/8(output8) -> or8/1
  VCU1_TorqueRef/1(output1) -> or1/2
  VCU1_TorqueRef/2(output2) -> or2/2
  VCU1_TorqueRef/3(output3) -> or3/2
  VCU1_TorqueRef/4(output4) -> or4/2
  VCU1_TorqueRef/5(output5) -> or5/2
  VCU1_TorqueRef/6(output6) -> or6/2
  VCU1_TorqueRef/7(output7) -> or7/2
  VCU1_TorqueRef/8(output8) -> or8/2
  VCU1_SpeedMax/1(output1) -> or1/3
  VCU1_SpeedMax/2(output2) -> or2/3
  VCU1_SpeedMax/3(output3) -> or3/3
  VCU1_SpeedMax/4(output4) -> or4/3
  VCU1_SpeedMax/5(output5) -> or5/3
  VCU1_SpeedMax/6(output6) -> or6/3
  VCU1_SpeedMax/7(output7) -> or7/3
  VCU1_SpeedMax/8(output8) -> or8/3
  VCU1_GearCmd/1(output1) -> or1/4
  VCU1_GearCmd/2(output2) -> or2/4
  VCU1_GearCmd/3(output3) -> or3/4
  VCU1_GearCmd/4(output4) -> or4/4
  VCU1_GearCmd/5(output5) -> or5/4
  VCU1_GearCmd/6(output6) -> or6/4
  VCU1_GearCmd/7(output7) -> or7/4
  VCU1_GearCmd/8(output8) -> or8/4
  VCU1_CtrlModel/1(output1) -> or1/5
  VCU1_CtrlModel/2(output2) -> or2/5
  VCU1_CtrlModel/3(output3) -> or3/5
  VCU1_CtrlModel/4(output4) -> or4/5
  VCU1_CtrlModel/5(output5) -> or5/5
  VCU1_CtrlModel/6(output6) -> or6/5
  VCU1_CtrlModel/7(output7) -> or7/5
  VCU1_CtrlModel/8(output8) -> or8/5
  VCU1_EnableReq/1(output1) -> or1/6
  VCU1_EnableReq/2(output2) -> or2/6
  VCU1_EnableReq/3(output3) -> or3/6
  VCU1_EnableReq/4(output4) -> or4/6
  VCU1_EnableReq/5(output5) -> or5/6
  VCU1_EnableReq/6(output6) -> or6/6
  VCU1_EnableReq/7(output7) -> or7/6
  VCU1_EnableReq/8(output8) -> or8/6
  or1/1 -> Conv1/1
  Conv1/1 -> VCU1_mux/1
  or2/1 -> Conv2/1
  Conv2/1 -> VCU1_mux/2
  or3/1 -> Conv3/1
  Conv3/1 -> VCU1_mux/3
  or4/1 -> Conv4/1
  Conv4/1 -> VCU1_mux/4
  or5/1 -> Conv5/1
  Conv5/1 -> VCU1_mux/5
  or6/1 -> Conv6/1
  Conv6/1 -> VCU1_mux/6
  or7/1 -> Conv7/1
  Conv7/1 -> VCU1_mux/7
  or8/1 -> Conv8/1
  Conv8/1 -> VCU1_mux/8
  VCU1_ID/1 -> VCU1_ID_Out/1
  VCU1_DLC/1 -> VCU1_DLC_Out/1
  VCU1_LifeCnt_in/1 -> VCU1_LifeCnt/1(VCU1_LifeCnt)
  VCU1_TorqueRef_in/1 -> VCU1_TorqueRef/1(VCU1_TorqueRef)
  VCU1_SpeedMax_in/1 -> VCU1_SpeedMax/1(VCU1_SpeedMax)
  VCU1_GearCmd_in/1 -> VCU1_GearCmd/1(VCU1_GearCmd)
  VCU1_CtrlModel_in/1 -> VCU1_CtrlModel/1(VCU1_CtrlModel)
  VCU1_EnableReq_in/1 -> VCU1_EnableReq/1(VCU1_EnableReq)

== system six_plus_six_AcmsteeringV09_main/Subsystem/VCU3 ==
  VCU1_EnableReq_in : Inport
  VCU1_CtrlModel_in : Inport  Port=2
  VCU1_GearCmd_in : Inport  Port=3
  VCU1_SpeedMax_in : Inport  Port=4
  VCU1_TorqueRef_in : Inport  Port=5
  VCU1_LifeCnt_in : Inport  Port=6
  Conv{1..8} (8 alike) : DataTypeConversion
  VCU1_CtrlModel : Subsystem
  VCU1_DLC : Constant  Value=8  OutDataTypeStr=uint8
  VCU1_DLC_Out : Terminator
  VCU1_EnableReq : Subsystem
  VCU1_GearCmd : Subsystem
  VCU1_ID : Constant  Value=2353065767  OutDataTypeStr=single
  VCU1_ID_Out : Terminator
  VCU1_LifeCnt : Subsystem
  VCU1_SpeedMax : Subsystem
  VCU1_TorqueRef : Subsystem
  VCU1_mux : Mux  Inputs=8
  or{1..8} (8 alike) : simulink/Logic and Bit Operations/Bitwise Operator  logicop=OR  UseBitMask=off  NumInputPorts=6  BitMask=bin2dec('11011001')  BitMaskRealWorld=Stored Integer
  output : Outport
  wires:
  VCU1_mux/1 -> output/1
  VCU1_LifeCnt/1(output1) -> or1/1
  VCU1_LifeCnt/2(output2) -> or2/1
  VCU1_LifeCnt/3(output3) -> or3/1
  VCU1_LifeCnt/4(output4) -> or4/1
  VCU1_LifeCnt/5(output5) -> or5/1
  VCU1_LifeCnt/6(output6) -> or6/1
  VCU1_LifeCnt/7(output7) -> or7/1
  VCU1_LifeCnt/8(output8) -> or8/1
  VCU1_TorqueRef/1(output1) -> or1/2
  VCU1_TorqueRef/2(output2) -> or2/2
  VCU1_TorqueRef/3(output3) -> or3/2
  VCU1_TorqueRef/4(output4) -> or4/2
  VCU1_TorqueRef/5(output5) -> or5/2
  VCU1_TorqueRef/6(output6) -> or6/2
  VCU1_TorqueRef/7(output7) -> or7/2
  VCU1_TorqueRef/8(output8) -> or8/2
  VCU1_SpeedMax/1(output1) -> or1/3
  VCU1_SpeedMax/2(output2) -> or2/3
  VCU1_SpeedMax/3(output3) -> or3/3
  VCU1_SpeedMax/4(output4) -> or4/3
  VCU1_SpeedMax/5(output5) -> or5/3
  VCU1_SpeedMax/6(output6) -> or6/3
  VCU1_SpeedMax/7(output7) -> or7/3
  VCU1_SpeedMax/8(output8) -> or8/3
  VCU1_GearCmd/1(output1) -> or1/4
  VCU1_GearCmd/2(output2) -> or2/4
  VCU1_GearCmd/3(output3) -> or3/4
  VCU1_GearCmd/4(output4) -> or4/4
  VCU1_GearCmd/5(output5) -> or5/4
  VCU1_GearCmd/6(output6) -> or6/4
  VCU1_GearCmd/7(output7) -> or7/4
  VCU1_GearCmd/8(output8) -> or8/4
  VCU1_CtrlModel/1(output1) -> or1/5
  VCU1_CtrlModel/2(output2) -> or2/5
  VCU1_CtrlModel/3(output3) -> or3/5
  VCU1_CtrlModel/4(output4) -> or4/5
  VCU1_CtrlModel/5(output5) -> or5/5
  VCU1_CtrlModel/6(output6) -> or6/5
  VCU1_CtrlModel/7(output7) -> or7/5
  VCU1_CtrlModel/8(output8) -> or8/5
  VCU1_EnableReq/1(output1) -> or1/6
  VCU1_EnableReq/2(output2) -> or2/6
  VCU1_EnableReq/3(output3) -> or3/6
  VCU1_EnableReq/4(output4) -> or4/6
  VCU1_EnableReq/5(output5) -> or5/6
  VCU1_EnableReq/6(output6) -> or6/6
  VCU1_EnableReq/7(output7) -> or7/6
  VCU1_EnableReq/8(output8) -> or8/6
  or1/1 -> Conv1/1
  Conv1/1 -> VCU1_mux/1
  or2/1 -> Conv2/1
  Conv2/1 -> VCU1_mux/2
  or3/1 -> Conv3/1
  Conv3/1 -> VCU1_mux/3
  or4/1 -> Conv4/1
  Conv4/1 -> VCU1_mux/4
  or5/1 -> Conv5/1
  Conv5/1 -> VCU1_mux/5
  or6/1 -> Conv6/1
  Conv6/1 -> VCU1_mux/6
  or7/1 -> Conv7/1
  Conv7/1 -> VCU1_mux/7
  or8/1 -> Conv8/1
  Conv8/1 -> VCU1_mux/8
  VCU1_ID/1 -> VCU1_ID_Out/1
  VCU1_DLC/1 -> VCU1_DLC_Out/1
  VCU1_LifeCnt_in/1 -> VCU1_LifeCnt/1(VCU1_LifeCnt)
  VCU1_TorqueRef_in/1 -> VCU1_TorqueRef/1(VCU1_TorqueRef)
  VCU1_SpeedMax_in/1 -> VCU1_SpeedMax/1(VCU1_SpeedMax)
  VCU1_GearCmd_in/1 -> VCU1_GearCmd/1(VCU1_GearCmd)
  VCU1_CtrlModel_in/1 -> VCU1_CtrlModel/1(VCU1_CtrlModel)
  VCU1_EnableReq_in/1 -> VCU1_EnableReq/1(VCU1_EnableReq)

== system six_plus_six_AcmsteeringV09_main/Subsystem/VCU4 ==
  VCU1_EnableReq_in : Inport
  VCU1_CtrlModel_in : Inport  Port=2
  VCU1_GearCmd_in : Inport  Port=3
  VCU1_SpeedMax_in : Inport  Port=4
  VCU1_TorqueRef_in : Inport  Port=5
  VCU1_LifeCnt_in : Inport  Port=6
  Conv{1..8} (8 alike) : DataTypeConversion
  VCU1_CtrlModel : Subsystem
  VCU1_DLC : Constant  Value=8  OutDataTypeStr=uint8
  VCU1_DLC_Out : Terminator
  VCU1_EnableReq : Subsystem
  VCU1_GearCmd : Subsystem
  VCU1_ID : Constant  Value=2353065767  OutDataTypeStr=single
  VCU1_ID_Out : Terminator
  VCU1_LifeCnt : Subsystem
  VCU1_SpeedMax : Subsystem
  VCU1_TorqueRef : Subsystem
  VCU1_mux : Mux  Inputs=8
  or{1..8} (8 alike) : simulink/Logic and Bit Operations/Bitwise Operator  logicop=OR  UseBitMask=off  NumInputPorts=6  BitMask=bin2dec('11011001')  BitMaskRealWorld=Stored Integer
  output : Outport
  wires:
  VCU1_mux/1 -> output/1
  VCU1_LifeCnt/1(output1) -> or1/1
  VCU1_LifeCnt/2(output2) -> or2/1
  VCU1_LifeCnt/3(output3) -> or3/1
  VCU1_LifeCnt/4(output4) -> or4/1
  VCU1_LifeCnt/5(output5) -> or5/1
  VCU1_LifeCnt/6(output6) -> or6/1
  VCU1_LifeCnt/7(output7) -> or7/1
  VCU1_LifeCnt/8(output8) -> or8/1
  VCU1_TorqueRef/1(output1) -> or1/2
  VCU1_TorqueRef/2(output2) -> or2/2
  VCU1_TorqueRef/3(output3) -> or3/2
  VCU1_TorqueRef/4(output4) -> or4/2
  VCU1_TorqueRef/5(output5) -> or5/2
  VCU1_TorqueRef/6(output6) -> or6/2
  VCU1_TorqueRef/7(output7) -> or7/2
  VCU1_TorqueRef/8(output8) -> or8/2
  VCU1_SpeedMax/1(output1) -> or1/3
  VCU1_SpeedMax/2(output2) -> or2/3
  VCU1_SpeedMax/3(output3) -> or3/3
  VCU1_SpeedMax/4(output4) -> or4/3
  VCU1_SpeedMax/5(output5) -> or5/3
  VCU1_SpeedMax/6(output6) -> or6/3
  VCU1_SpeedMax/7(output7) -> or7/3
  VCU1_SpeedMax/8(output8) -> or8/3
  VCU1_GearCmd/1(output1) -> or1/4
  VCU1_GearCmd/2(output2) -> or2/4
  VCU1_GearCmd/3(output3) -> or3/4
  VCU1_GearCmd/4(output4) -> or4/4
  VCU1_GearCmd/5(output5) -> or5/4
  VCU1_GearCmd/6(output6) -> or6/4
  VCU1_GearCmd/7(output7) -> or7/4
  VCU1_GearCmd/8(output8) -> or8/4
  VCU1_CtrlModel/1(output1) -> or1/5
  VCU1_CtrlModel/2(output2) -> or2/5
  VCU1_CtrlModel/3(output3) -> or3/5
  VCU1_CtrlModel/4(output4) -> or4/5
  VCU1_CtrlModel/5(output5) -> or5/5
  VCU1_CtrlModel/6(output6) -> or6/5
  VCU1_CtrlModel/7(output7) -> or7/5
  VCU1_CtrlModel/8(output8) -> or8/5
  VCU1_EnableReq/1(output1) -> or1/6
  VCU1_EnableReq/2(output2) -> or2/6
  VCU1_EnableReq/3(output3) -> or3/6
  VCU1_EnableReq/4(output4) -> or4/6
  VCU1_EnableReq/5(output5) -> or5/6
  VCU1_EnableReq/6(output6) -> or6/6
  VCU1_EnableReq/7(output7) -> or7/6
  VCU1_EnableReq/8(output8) -> or8/6
  or1/1 -> Conv1/1
  Conv1/1 -> VCU1_mux/1
  or2/1 -> Conv2/1
  Conv2/1 -> VCU1_mux/2
  or3/1 -> Conv3/1
  Conv3/1 -> VCU1_mux/3
  or4/1 -> Conv4/1
  Conv4/1 -> VCU1_mux/4
  or5/1 -> Conv5/1
  Conv5/1 -> VCU1_mux/5
  or6/1 -> Conv6/1
  Conv6/1 -> VCU1_mux/6
  or7/1 -> Conv7/1
  Conv7/1 -> VCU1_mux/7
  or8/1 -> Conv8/1
  Conv8/1 -> VCU1_mux/8
  VCU1_ID/1 -> VCU1_ID_Out/1
  VCU1_DLC/1 -> VCU1_DLC_Out/1
  VCU1_LifeCnt_in/1 -> VCU1_LifeCnt/1(VCU1_LifeCnt)
  VCU1_TorqueRef_in/1 -> VCU1_TorqueRef/1(VCU1_TorqueRef)
  VCU1_SpeedMax_in/1 -> VCU1_SpeedMax/1(VCU1_SpeedMax)
  VCU1_GearCmd_in/1 -> VCU1_GearCmd/1(VCU1_GearCmd)
  VCU1_CtrlModel_in/1 -> VCU1_CtrlModel/1(VCU1_CtrlModel)
  VCU1_EnableReq_in/1 -> VCU1_EnableReq/1(VCU1_EnableReq)

== system six_plus_six_AcmsteeringV09_main/Subsystem/VCU5 ==
  VCU1_EnableReq_in : Inport
  VCU1_CtrlModel_in : Inport  Port=2
  VCU1_GearCmd_in : Inport  Port=3
  VCU1_SpeedMax_in : Inport  Port=4
  VCU1_TorqueRef_in : Inport  Port=5
  VCU1_LifeCnt_in : Inport  Port=6
  Conv{1..8} (8 alike) : DataTypeConversion
  VCU1_CtrlModel : Subsystem
  VCU1_DLC : Constant  Value=8  OutDataTypeStr=uint8
  VCU1_DLC_Out : Terminator
  VCU1_EnableReq : Subsystem
  VCU1_GearCmd : Subsystem
  VCU1_ID : Constant  Value=2353065767  OutDataTypeStr=single
  VCU1_ID_Out : Terminator
  VCU1_LifeCnt : Subsystem
  VCU1_SpeedMax : Subsystem
  VCU1_TorqueRef : Subsystem
  VCU1_mux : Mux  Inputs=8
  or{1..8} (8 alike) : simulink/Logic and Bit Operations/Bitwise Operator  logicop=OR  UseBitMask=off  NumInputPorts=6  BitMask=bin2dec('11011001')  BitMaskRealWorld=Stored Integer
  output : Outport
  wires:
  VCU1_mux/1 -> output/1
  VCU1_LifeCnt/1(output1) -> or1/1
  VCU1_LifeCnt/2(output2) -> or2/1
  VCU1_LifeCnt/3(output3) -> or3/1
  VCU1_LifeCnt/4(output4) -> or4/1
  VCU1_LifeCnt/5(output5) -> or5/1
  VCU1_LifeCnt/6(output6) -> or6/1
  VCU1_LifeCnt/7(output7) -> or7/1
  VCU1_LifeCnt/8(output8) -> or8/1
  VCU1_TorqueRef/1(output1) -> or1/2
  VCU1_TorqueRef/2(output2) -> or2/2
  VCU1_TorqueRef/3(output3) -> or3/2
  VCU1_TorqueRef/4(output4) -> or4/2
  VCU1_TorqueRef/5(output5) -> or5/2
  VCU1_TorqueRef/6(output6) -> or6/2
  VCU1_TorqueRef/7(output7) -> or7/2
  VCU1_TorqueRef/8(output8) -> or8/2
  VCU1_SpeedMax/1(output1) -> or1/3
  VCU1_SpeedMax/2(output2) -> or2/3
  VCU1_SpeedMax/3(output3) -> or3/3
  VCU1_SpeedMax/4(output4) -> or4/3
  VCU1_SpeedMax/5(output5) -> or5/3
  VCU1_SpeedMax/6(output6) -> or6/3
  VCU1_SpeedMax/7(output7) -> or7/3
  VCU1_SpeedMax/8(output8) -> or8/3
  VCU1_GearCmd/1(output1) -> or1/4
  VCU1_GearCmd/2(output2) -> or2/4
  VCU1_GearCmd/3(output3) -> or3/4
  VCU1_GearCmd/4(output4) -> or4/4
  VCU1_GearCmd/5(output5) -> or5/4
  VCU1_GearCmd/6(output6) -> or6/4
  VCU1_GearCmd/7(output7) -> or7/4
  VCU1_GearCmd/8(output8) -> or8/4
  VCU1_CtrlModel/1(output1) -> or1/5
  VCU1_CtrlModel/2(output2) -> or2/5
  VCU1_CtrlModel/3(output3) -> or3/5
  VCU1_CtrlModel/4(output4) -> or4/5
  VCU1_CtrlModel/5(output5) -> or5/5
  VCU1_CtrlModel/6(output6) -> or6/5
  VCU1_CtrlModel/7(output7) -> or7/5
  VCU1_CtrlModel/8(output8) -> or8/5
  VCU1_EnableReq/1(output1) -> or1/6
  VCU1_EnableReq/2(output2) -> or2/6
  VCU1_EnableReq/3(output3) -> or3/6
  VCU1_EnableReq/4(output4) -> or4/6
  VCU1_EnableReq/5(output5) -> or5/6
  VCU1_EnableReq/6(output6) -> or6/6
  VCU1_EnableReq/7(output7) -> or7/6
  VCU1_EnableReq/8(output8) -> or8/6
  or1/1 -> Conv1/1
  Conv1/1 -> VCU1_mux/1
  or2/1 -> Conv2/1
  Conv2/1 -> VCU1_mux/2
  or3/1 -> Conv3/1
  Conv3/1 -> VCU1_mux/3
  or4/1 -> Conv4/1
  Conv4/1 -> VCU1_mux/4
  or5/1 -> Conv5/1
  Conv5/1 -> VCU1_mux/5
  or6/1 -> Conv6/1
  Conv6/1 -> VCU1_mux/6
  or7/1 -> Conv7/1
  Conv7/1 -> VCU1_mux/7
  or8/1 -> Conv8/1
  Conv8/1 -> VCU1_mux/8
  VCU1_ID/1 -> VCU1_ID_Out/1
  VCU1_DLC/1 -> VCU1_DLC_Out/1
  VCU1_LifeCnt_in/1 -> VCU1_LifeCnt/1(VCU1_LifeCnt)
  VCU1_TorqueRef_in/1 -> VCU1_TorqueRef/1(VCU1_TorqueRef)
  VCU1_SpeedMax_in/1 -> VCU1_SpeedMax/1(VCU1_SpeedMax)
  VCU1_GearCmd_in/1 -> VCU1_GearCmd/1(VCU1_GearCmd)
  VCU1_CtrlModel_in/1 -> VCU1_CtrlModel/1(VCU1_CtrlModel)
  VCU1_EnableReq_in/1 -> VCU1_EnableReq/1(VCU1_EnableReq)

== system six_plus_six_AcmsteeringV09_main/Subsystem/VCU6 ==
  VCU1_EnableReq_in : Inport
  VCU1_CtrlModel_in : Inport  Port=2
  VCU1_GearCmd_in : Inport  Port=3
  VCU1_SpeedMax_in : Inport  Port=4
  VCU1_TorqueRef_in : Inport  Port=5
  VCU1_LifeCnt_in : Inport  Port=6
  Conv{1..8} (8 alike) : DataTypeConversion
  VCU1_CtrlModel : Subsystem
  VCU1_DLC : Constant  Value=8  OutDataTypeStr=uint8
  VCU1_DLC_Out : Terminator
  VCU1_EnableReq : Subsystem
  VCU1_GearCmd : Subsystem
  VCU1_ID : Constant  Value=2353065767  OutDataTypeStr=single
  VCU1_ID_Out : Terminator
  VCU1_LifeCnt : Subsystem
  VCU1_SpeedMax : Subsystem
  VCU1_TorqueRef : Subsystem
  VCU1_mux : Mux  Inputs=8
  or{1..8} (8 alike) : simulink/Logic and Bit Operations/Bitwise Operator  logicop=OR  UseBitMask=off  NumInputPorts=6  BitMask=bin2dec('11011001')  BitMaskRealWorld=Stored Integer
  output : Outport
  wires:
  VCU1_mux/1 -> output/1
  VCU1_LifeCnt/1(output1) -> or1/1
  VCU1_LifeCnt/2(output2) -> or2/1
  VCU1_LifeCnt/3(output3) -> or3/1
  VCU1_LifeCnt/4(output4) -> or4/1
  VCU1_LifeCnt/5(output5) -> or5/1
  VCU1_LifeCnt/6(output6) -> or6/1
  VCU1_LifeCnt/7(output7) -> or7/1
  VCU1_LifeCnt/8(output8) -> or8/1
  VCU1_TorqueRef/1(output1) -> or1/2
  VCU1_TorqueRef/2(output2) -> or2/2
  VCU1_TorqueRef/3(output3) -> or3/2
  VCU1_TorqueRef/4(output4) -> or4/2
  VCU1_TorqueRef/5(output5) -> or5/2
  VCU1_TorqueRef/6(output6) -> or6/2
  VCU1_TorqueRef/7(output7) -> or7/2
  VCU1_TorqueRef/8(output8) -> or8/2
  VCU1_SpeedMax/1(output1) -> or1/3
  VCU1_SpeedMax/2(output2) -> or2/3
  VCU1_SpeedMax/3(output3) -> or3/3
  VCU1_SpeedMax/4(output4) -> or4/3
  VCU1_SpeedMax/5(output5) -> or5/3
  VCU1_SpeedMax/6(output6) -> or6/3
  VCU1_SpeedMax/7(output7) -> or7/3
  VCU1_SpeedMax/8(output8) -> or8/3
  VCU1_GearCmd/1(output1) -> or1/4
  VCU1_GearCmd/2(output2) -> or2/4
  VCU1_GearCmd/3(output3) -> or3/4
  VCU1_GearCmd/4(output4) -> or4/4
  VCU1_GearCmd/5(output5) -> or5/4
  VCU1_GearCmd/6(output6) -> or6/4
  VCU1_GearCmd/7(output7) -> or7/4
  VCU1_GearCmd/8(output8) -> or8/4
  VCU1_CtrlModel/1(output1) -> or1/5
  VCU1_CtrlModel/2(output2) -> or2/5
  VCU1_CtrlModel/3(output3) -> or3/5
  VCU1_CtrlModel/4(output4) -> or4/5
  VCU1_CtrlModel/5(output5) -> or5/5
  VCU1_CtrlModel/6(output6) -> or6/5
  VCU1_CtrlModel/7(output7) -> or7/5
  VCU1_CtrlModel/8(output8) -> or8/5
  VCU1_EnableReq/1(output1) -> or1/6
  VCU1_EnableReq/2(output2) -> or2/6
  VCU1_EnableReq/3(output3) -> or3/6
  VCU1_EnableReq/4(output4) -> or4/6
  VCU1_EnableReq/5(output5) -> or5/6
  VCU1_EnableReq/6(output6) -> or6/6
  VCU1_EnableReq/7(output7) -> or7/6
  VCU1_EnableReq/8(output8) -> or8/6
  or1/1 -> Conv1/1
  Conv1/1 -> VCU1_mux/1
  or2/1 -> Conv2/1
  Conv2/1 -> VCU1_mux/2
  or3/1 -> Conv3/1
  Conv3/1 -> VCU1_mux/3
  or4/1 -> Conv4/1
  Conv4/1 -> VCU1_mux/4
  or5/1 -> Conv5/1
  Conv5/1 -> VCU1_mux/5
  or6/1 -> Conv6/1
  Conv6/1 -> VCU1_mux/6
  or7/1 -> Conv7/1
  Conv7/1 -> VCU1_mux/7
  or8/1 -> Conv8/1
  Conv8/1 -> VCU1_mux/8
  VCU1_ID/1 -> VCU1_ID_Out/1
  VCU1_DLC/1 -> VCU1_DLC_Out/1
  VCU1_LifeCnt_in/1 -> VCU1_LifeCnt/1(VCU1_LifeCnt)
  VCU1_TorqueRef_in/1 -> VCU1_TorqueRef/1(VCU1_TorqueRef)
  VCU1_SpeedMax_in/1 -> VCU1_SpeedMax/1(VCU1_SpeedMax)
  VCU1_GearCmd_in/1 -> VCU1_GearCmd/1(VCU1_GearCmd)
  VCU1_CtrlModel_in/1 -> VCU1_CtrlModel/1(VCU1_CtrlModel)
  VCU1_EnableReq_in/1 -> VCU1_EnableReq/1(VCU1_EnableReq)

== system six_plus_six_AcmsteeringV09_main/Data_input/1/Enabled Subsystem ==
  In2 : Inport
  Enable : EnablePort
  Add : Sum
  Constant : Constant  Value=256
  Constant1 : Constant  SampleTime=-1
  Constant3 : Constant  Value=256
  Data Type Conversion{8..13} (6 alike) : DataTypeConversion  OutDataTypeStr=uint8
  Demux1 : Demux  Outputs=6
  MATLAB Function1 : MATLAB Function  TreatAsAtomicUnit=on
  MATLAB Function3 : MATLAB Function  TreatAsAtomicUnit=on
  Memory : Memory  InheritSampleTime=on
  Product : Product
  Product2 : Product
  Saturation : Saturate  UpperLimit=5  LowerLimit=0
  Sum : Sum  Inputs=|++
  Sum1 : Sum  Inputs=|++
  Terminator1 : Terminator
  Terminator2 : Terminator
  motec_spd_2 : Outport
  motec_current_2 : Outport  Port=2
  enable_count2 : Outport  Port=3
  wires:
  In2/1 -> Demux1/1
  Demux1/1 -> Data Type Conversion8/1
  Demux1/2 -> Data Type Conversion9/1
  Demux1/3 -> Data Type Conversion10/1
  Demux1/4 -> Data Type Conversion11/1
  Demux1/5 -> Data Type Conversion13/1
  Demux1/6 -> Data Type Conversion12/1
  Data Type Conversion8/1 -> Terminator1/1
  Data Type Conversion9/1 -> Terminator2/1
  Data Type Conversion10/1 -> Sum/1
  Data Type Conversion11/1 -> Product/2
  Constant/1 -> Product/1
  Product/1 -> Sum/2
  Sum/1 -> MATLAB Function3/1(speed)
  Data Type Conversion12/1 -> Product2/2
  Constant3/1 -> Product2/1
  Product2/1 -> Sum1/2
  Data Type Conversion13/1 -> Sum1/1
  Sum1/1 -> MATLAB Function1/1(current_in)
  MATLAB Function3/1(speed_out) -> motec_spd_2/1
  MATLAB Function1/1(current_out) -> motec_current_2/1
  Constant1/1 -> Add/1
  Memory/1 -> Add/2
  Add/1 -> Saturation/1
  Saturation/1 -> enable_count2/1, Memory/1

== system six_plus_six_AcmsteeringV09_main/Data_input/10/Enabled Subsystem ==
  In2 : Inport
  Enable : EnablePort
  Data Type Conversion{,1..7} (8 alike) : DataTypeConversion
  Demux1 : Demux  Outputs=8
  MATLAB Function : MATLAB Function  TreatAsAtomicUnit=on
  MATLAB Function1 : MATLAB Function  TreatAsAtomicUnit=on
  Rolling_Out : Outport
  Heading_Out : Outport  Port=2
  wires:
  Demux1/8 -> Data Type Conversion3/1
  Demux1/7 -> Data Type Conversion2/1
  Demux1/6 -> Data Type Conversion1/1
  Demux1/5 -> Data Type Conversion/1
  MATLAB Function1/1(y) -> Heading_Out/1
  MATLAB Function/1(y) -> Rolling_Out/1
  Demux1/1 -> Data Type Conversion4/1
  Demux1/2 -> Data Type Conversion5/1
  Demux1/3 -> Data Type Conversion6/1
  Demux1/4 -> Data Type Conversion7/1
  In2/1 -> Demux1/1
  Data Type Conversion/1 -> MATLAB Function1/1(data1)
  Data Type Conversion1/1 -> MATLAB Function1/2(data2)
  Data Type Conversion2/1 -> MATLAB Function1/3(data3)
  Data Type Conversion3/1 -> MATLAB Function1/4(data4)
  Data Type Conversion4/1 -> MATLAB Function/1(data1)
  Data Type Conversion5/1 -> MATLAB Function/2(data2)
  Data Type Conversion6/1 -> MATLAB Function/3(data3)
  Data Type Conversion7/1 -> MATLAB Function/4(data4)
